simulink model "Battery"  (R2025b)
settings: Solver=VariableStepAuto  StartTime=0.0  StopTime=100  MaxStep=0.01  RelTol=1e-3
undefined symbols (not defined in the file or in its folder): Cn, I, OCV, R_Charge, R_Discharge, SOC
settings Model: Creator=night  LastModifiedBy=night

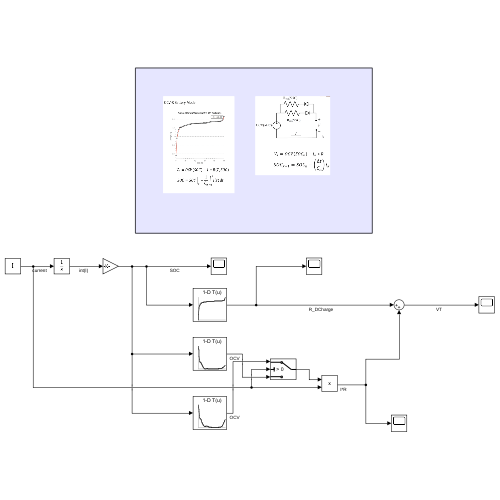
[thumbnail: Simulink's stored preview of the top-level diagram]
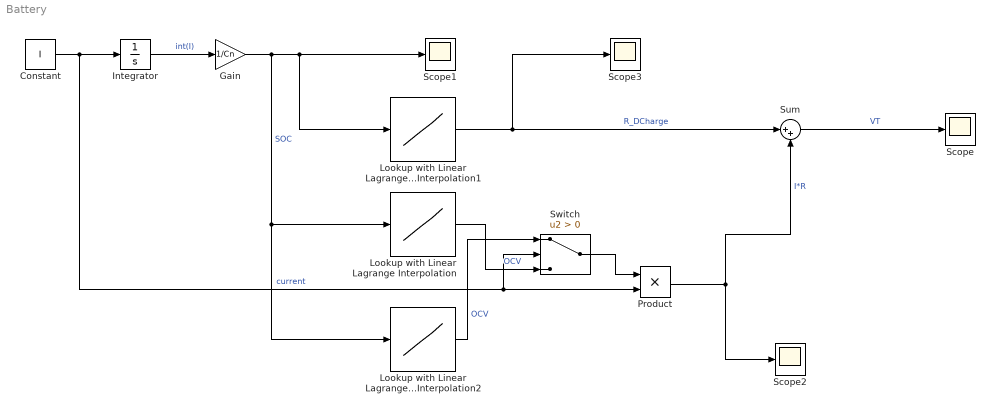
== system Battery ==
  Constant : Constant  Value=I
  Gain : Gain  Gain=1/Cn
  Integrator : Integrator
  Lookup with Linear Lagrange Interpolation : Lookup_n-D  NumberOfTableDimensions=1  BreakpointsForDimension1=SOC  Table=R_Discharge  InterpMethod=Linear Lagrange  InternalRulePriority=Speed  RndMeth=Simplest
  Lookup with Linear Lagrange Interpolation1 : Lookup_n-D  NumberOfTableDimensions=1  BreakpointsForDimension1=SOC  Table=OCV  InterpMethod=Linear Lagrange  InternalRulePriority=Speed  RndMeth=Simplest
  Lookup with Linear Lagrange Interpolation2 : Lookup_n-D  NumberOfTableDimensions=1  BreakpointsForDimension1=SOC  Table=R_Charge  InterpMethod=Linear Lagrange  InternalRulePriority=Speed  RndMeth=Simplest
  Product : Product
  Scope{,1..3} (4 alike) : Scope
      Scope settings: TimeSpan=1  ActiveDisplayYMinimum=2.5431799999999987  ActiveDisplayYMaximum=4.7913800000000135
      Scope1 settings: ActiveDisplayYMinimum=-0.12500000000000008  ActiveDisplayYMaximum=1.1250000000000009
      Scope2 settings: ActiveDisplayYMinimum=0.0700391304347826  ActiveDisplayYMaximum=0.1699956521739131  DataLoggingVariableName=ScopeData2
      Scope3 settings: ActiveDisplayYMinimum=-1  ActiveDisplayYMaximum=1  DataLoggingVariableName=ScopeData3
  Sum : Sum  Inputs=|++
  Switch : Switch  Criteria=u2 > Threshold  SaturateOnIntegerOverflow=off  InputSameDT=off
  wires:
  Constant/1 -> Switch/2, Product/2, Integrator/1  "current"
  Integrator/1 -> Gain/1  "int(I)"
  Gain/1 -> Lookup with Linear Lagrange Interpolation1/1, Scope1/1, Lookup with Linear Lagrange Interpolation2/1, Lookup with Linear Lagrange Interpolation/1  "SOC"
  Lookup with Linear Lagrange Interpolation1/1 -> Scope3/1, Sum/1  "R_DCharge"
  Product/1 -> Sum/2, Scope2/1  "I*R"
  Sum/1 -> Scope/1  "VT"
  Lookup with Linear Lagrange Interpolation/1 -> Switch/3  "OCV"
  Lookup with Linear Lagrange Interpolation2/1 -> Switch/1  "OCV"
  Switch/1 -> Product/1
